simulink model "Controller_Design"  (R2018b)
settings: Solver=VariableStepAuto  StartTime=0.0  StopTime=7000  RelTol=1e-3
values from neighbouring files (symbols this model uses):
  kd = 0.01375    [ControllerDesign.m]
  ki = ki    [ControllerDesign.m]
  kprop = kprop    [ControllerDesign.m]
libraries: cstblocks x4, simulink x3
settings Model: Creator=lenovo  LastModifiedBy=lenovo
settings DataIOCC: MaxDataPoints=10000  DSMLogging=off
settings CodeAppCC: StateflowObjectComments=on

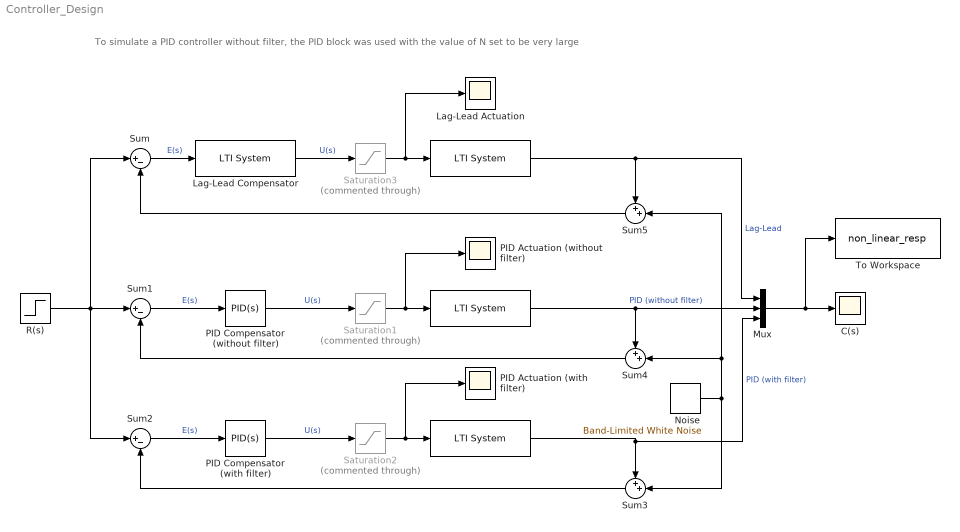
== system Controller_Design ==
  note: To simulate a PID controller without filter, the PID block was used with the value of N set to be very large
  " " : cstblocks/LTI System  sys=G2  IC=[]
  "  " : cstblocks/LTI System  sys=G2  IC=[]
  "      " : cstblocks/LTI System  sys=G2  IC=[]
  C(s) : Scope
  Lag-Lead Actuation : Scope
  Lag-Lead Compensator : cstblocks/LTI System  sys=G_lag_lead  IC=[]
  Mux : Mux  Inputs=3
  Noise : simulink/Sources/Band-Limited White Noise  Cov=0.1  Ts=1  seed=[23341]
  PID Actuation (with filter) : Scope
  PID Actuation (without filter) : Scope
  "PID Compensator (with filter) " : simulink/Continuous/PID Controller  Controller=PID  Form=Parallel  TimeDomain=Continuous-time  SampleTime=-1  IntegratorMethod=Forward Euler  FilterMethod=Forward Euler  ControllerParametersSource=internal  P=kprop  I=ki  D=kd  UseFilter=on  N=1e-2  TunerSelectOption=Transfer Function Based (PID Tuner App)  InitialConditionSource=internal  InitialConditionForIntegrator=0  InitialConditionForFilter=0  DifferentiatorICPrevScaledInput=0  ExternalReset=none  TrackingMode=off  Kt=1  LimitOutput=off  UpperSaturationLimit=inf  LowerSaturationLimit=-inf  LinearizeAsGain=on  AntiWindupMode=none  Kb=1  POutMin=[]  POutMax=[]  IOutMin=[]  IOutMax=[]  DOutMin=[]  DOutMax=[]  NOutMin=[]  NOutMax=[]  SumOutMin=[]  SumOutMax=[]  SaturationOutMin=[]  SaturationOutMax=[]  PParamMin=[]  PParamMax=[]  IParamMin=[]  IParamMax=[]  DParamMin=[]  DParamMax=[]  NParamMin=[]  NParamMax=[]  KbParamMin=[]  KbParamMax=[]  KtParamMin=[]  KtParamMax=[]  KbOutMin=[]  KbOutMax=[]  KtOutMin=[]  KtOutMax=[]  IntegratorOutMin=[]  IntegratorOutMax=[]  FilterOutMin=[]  FilterOutMax=[]  SumI1OutMin=[]  SumI1OutMax=[]  SumI2OutMin=[]  SumI2OutMax=[]  SumI3OutMin=[]  SumI3OutMax=[]  SumI4OutMin=[]  SumI4OutMax=[]  SumDOutMin=[]  SumDOutMax=[]  DifferentiatorOutMin=[]  DifferentiatorOutMax=[]  FilterDiffOutCoefMin=[]  FilterDiffOutCoefMax=[]  ReciprocalOutMin=[]  ReciprocalOutMax=[]  SumDenOutMin=[]  SumDenOutMax=[]  SumNumOutMin=[]  SumNumOutMax=[]  DivideOutMin=[]  DivideOutMax=[]  IntegratorContinuousStateAttributes=''  IntegratorStateMustResolveToSignalObject=off  IntegratorRTWStateStorageClass=Auto  FilterContinuousStateAttributes=''  FilterStateMustResolveToSignalObject=off  FilterRTWStateStorageClass=Auto  ParallelPVariant=InternalParameters  IdealPVariant=Disabled  IVariant=InternalParameters  DVariant=InternalParameters  IntegratorVariant=Continuous  SatVariant=Disabled  AWVariant=Passthrough  PCopyVariant=Disabled  TRVariant=Disabled  FdbkBlocksVariant=Forward  IdealPFdbkVariant=Disabled  SatFdbkVariant=Disabled  DerivativeFilterVariant=ContFilter  NVariant=InternalParameters  NCopyVariant=Disabled  FilterICVariant=InternalICsFilter  IntegratorICVariant=InternalICs  ExternalResetVariant=Disabled  TRSumVariant=Passthrough  SumFdbkVariant=Disabled  SumVariant=Sum_PID
  "PID Compensator (without filter) " : simulink/Continuous/PID Controller  Controller=PID  Form=Parallel  TimeDomain=Continuous-time  SampleTime=-1  IntegratorMethod=Forward Euler  FilterMethod=Forward Euler  ControllerParametersSource=internal  P=kprop  I=ki  D=kd  UseFilter=on  N=10000000  TunerSelectOption=Transfer Function Based (PID Tuner App)  InitialConditionSource=internal  InitialConditionForIntegrator=0  InitialConditionForFilter=0  DifferentiatorICPrevScaledInput=0  ExternalReset=none  TrackingMode=off  Kt=1  LimitOutput=off  UpperSaturationLimit=inf  LowerSaturationLimit=-inf  LinearizeAsGain=on  AntiWindupMode=none  Kb=1  POutMin=[]  POutMax=[]  IOutMin=[]  IOutMax=[]  DOutMin=[]  DOutMax=[]  NOutMin=[]  NOutMax=[]  SumOutMin=[]  SumOutMax=[]  SaturationOutMin=[]  SaturationOutMax=[]  PParamMin=[]  PParamMax=[]  IParamMin=[]  IParamMax=[]  DParamMin=[]  DParamMax=[]  NParamMin=[]  NParamMax=[]  KbParamMin=[]  KbParamMax=[]  KtParamMin=[]  KtParamMax=[]  KbOutMin=[]  KbOutMax=[]  KtOutMin=[]  KtOutMax=[]  IntegratorOutMin=[]  IntegratorOutMax=[]  FilterOutMin=[]  FilterOutMax=[]  SumI1OutMin=[]  SumI1OutMax=[]  SumI2OutMin=[]  SumI2OutMax=[]  SumI3OutMin=[]  SumI3OutMax=[]  SumI4OutMin=[]  SumI4OutMax=[]  SumDOutMin=[]  SumDOutMax=[]  DifferentiatorOutMin=[]  DifferentiatorOutMax=[]  FilterDiffOutCoefMin=[]  FilterDiffOutCoefMax=[]  ReciprocalOutMin=[]  ReciprocalOutMax=[]  SumDenOutMin=[]  SumDenOutMax=[]  SumNumOutMin=[]  SumNumOutMax=[]  DivideOutMin=[]  DivideOutMax=[]  IntegratorContinuousStateAttributes=''  IntegratorStateMustResolveToSignalObject=off  IntegratorRTWStateStorageClass=Auto  FilterContinuousStateAttributes=''  FilterStateMustResolveToSignalObject=off  FilterRTWStateStorageClass=Auto  ParallelPVariant=InternalParameters  IdealPVariant=Disabled  IVariant=InternalParameters  DVariant=InternalParameters  IntegratorVariant=Continuous  SatVariant=Disabled  AWVariant=Passthrough  PCopyVariant=Disabled  TRVariant=Disabled  FdbkBlocksVariant=Forward  IdealPFdbkVariant=Disabled  SatFdbkVariant=Disabled  DerivativeFilterVariant=ContFilter  NVariant=InternalParameters  NCopyVariant=Disabled  FilterICVariant=InternalICsFilter  IntegratorICVariant=InternalICs  ExternalResetVariant=Disabled  TRSumVariant=Passthrough  SumFdbkVariant=Disabled  SumVariant=Sum_PID
  R(s) : Step  SampleTime=0
  Saturation1 : Saturate  Commented=through  UpperLimit=2e-5  LowerLimit=0  ZeroCross=off
  Saturation2 : Saturate  Commented=through  UpperLimit=2e-5  LowerLimit=0  ZeroCross=off
  Saturation3 : Saturate  Commented=through  UpperLimit=2e-5  LowerLimit=0  ZeroCross=off
  Sum : Sum  Inputs=|+-
  Sum1 : Sum  Inputs=|+-
  Sum2 : Sum  Inputs=|+-
  Sum3 : Sum  Inputs=++|
  Sum4 : Sum  Inputs=++|
  Sum5 : Sum  Inputs=++|
  To Workspace : ToWorkspace  VariableName=non_linear_resp  SaveFormat=Timeseries  SampleTime=-1
  wires:
  " "/1 -> Sum5/1, Mux/1  "Lag-Lead"
  Sum/1 -> Lag-Lead Compensator/1  "E(s)"
  Lag-Lead Compensator/1 -> Saturation3/1  "U(s)"
  "  "/1 -> Mux/2, Sum4/1  "PID (without filter)"
  Mux/1 -> To Workspace/1, C(s)/1
  R(s)/1 -> Sum/1, Sum1/1, Sum2/1
  "      "/1 -> Mux/3, Sum3/1  "PID (with filter)"
  Sum2/1 -> "PID Compensator (with filter) "/1  "E(s)"
  "PID Compensator (with filter) "/1 -> Saturation2/1  "U(s)"
  Sum3/1 -> Sum2/2
  Noise/1 -> Sum5/2, Sum4/2, Sum3/2
  Sum5/1 -> Sum/2
  "PID Compensator (without filter) "/1 -> Saturation1/1  "U(s)"
  Sum1/1 -> "PID Compensator (without filter) "/1  "E(s)"
  Sum4/1 -> Sum1/2
  Saturation1/1 -> "  "/1, PID Actuation (without filter)/1
  Saturation2/1 -> "      "/1, PID Actuation (with filter)/1
  Saturation3/1 -> Lag-Lead Actuation/1, " "/1
